simulink model "x1_2_P2_Control_Loop"  (R2021b)
settings: Solver=VariableStepAuto  StartTime=0.0  StopTime=2000  RelTol=1e-3
libraries: slpidlib x2
settings Model: Creator=Edwar  LastModifiedBy=Edwar

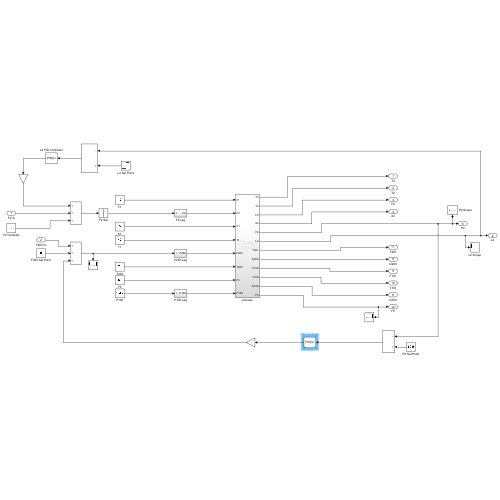
[thumbnail: Simulink's stored preview of the top-level diagram]
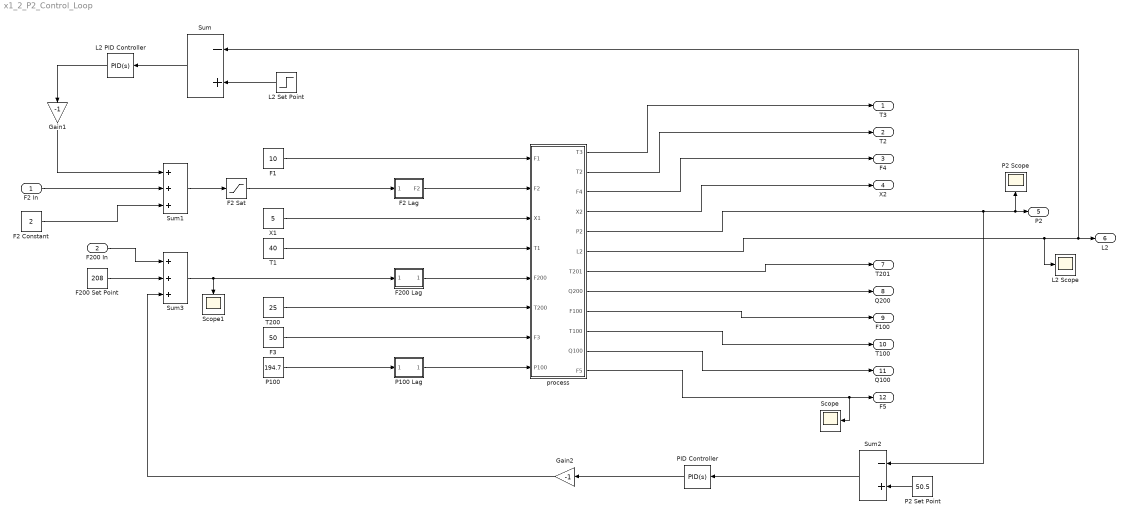
== system x1_2_P2_Control_Loop ==
  F2 In : Inport
  F200 In : Inport  Port=2
  F1 : Constant  Value=10
  F2 Constant : Constant  Value=2
  F2 Lag : Subsystem
  F2 Sat : Saturate  UpperLimit=4  LowerLimit=0
  F200 Lag : Subsystem
  F200 Set Point : Constant  Value=208
  F3 : Constant  Value=50
  Gain1 : Gain  Gain=-1
  Gain2 : Gain  Gain=-1
  L2 PID Controller : slpidlib/PID Controller  Controller=PID  Form=Ideal  TimeDomain=Continuous-time  UseExternalTs=off  SampleTime=-1  IntegratorMethod=Forward Euler  FilterMethod=Forward Euler  ControllerParametersSource=internal  P=14  I=1/19  D=0  UseFilter=on  N=100  TunerSelectOption=Transfer Function Based (PID Tuner App)  InitialConditionSource=internal  InitialConditionForIntegrator=0  InitialConditionForFilter=0  DifferentiatorICPrevScaledInput=0  ExternalReset=none  TrackingMode=off  Kt=1  LimitOutput=off  SatLimitsSource=internal  UpperSaturationLimit=inf  LowerSaturationLimit=-inf  LinearizeAsGain=on  AntiWindupMode=none  Kb=1  POutMin=[]  POutMax=[]  IOutMin=[]  IOutMax=[]  DOutMin=[]  DOutMax=[]  NOutMin=[]  NOutMax=[]  SumOutMin=[]  SumOutMax=[]  SaturationOutMin=[]  SaturationOutMax=[]  PParamMin=[]  PParamMax=[]  IParamMin=[]  IParamMax=[]  DParamMin=[]  DParamMax=[]  NParamMin=[]  NParamMax=[]  KbParamMin=[]  KbParamMax=[]  KtParamMin=[]  KtParamMax=[]  KbOutMin=[]  KbOutMax=[]  KtOutMin=[]  KtOutMax=[]  IntegratorOutMin=[]  IntegratorOutMax=[]  FilterOutMin=[]  FilterOutMax=[]  SumI1OutMin=[]  SumI1OutMax=[]  SumI2OutMin=[]  SumI2OutMax=[]  SumI3OutMin=[]  SumI3OutMax=[]  SumI4OutMin=[]  SumI4OutMax=[]  SumDOutMin=[]  SumDOutMax=[]  DifferentiatorOutMin=[]  DifferentiatorOutMax=[]  FilterDiffOutCoefMin=[]  FilterDiffOutCoefMax=[]  ReciprocalOutMin=[]  ReciprocalOutMax=[]  SumDenOutMin=[]  SumDenOutMax=[]  SumNumOutMin=[]  SumNumOutMax=[]  DivideOutMin=[]  DivideOutMax=[]  UdiffTsProdOutMin=[]  UdiffTsProdOutMax=[]  NTsProdOutMin=[]  NTsProdOutMax=[]  UintegralTsProdOutMin=[]  UintegralTsProdOutMax=[]  UngainTsProdOutMin=[]  UngainTsProdOutMax=[]  IntegratorContinuousStateAttributes=''  IntegratorStateMustResolveToSignalObject=off  IntegratorRTWStateStorageClass=Auto  FilterContinuousStateAttributes=''  FilterStateMustResolveToSignalObject=off  FilterRTWStateStorageClass=Auto  ParallelPVariant=Passthrough  IdealPVariant=InternalParameters  IVariant=InternalParameters  DVariant=InternalParameters  IntegratorVariant=Continuous  SatVariant=Disabled  AWVariant=Passthrough  PCopyVariant=Disabled  TRVariant=Disabled  FdbkBlocksVariant=Forward  IdealPFdbkVariant=Disabled  SatFdbkVariant=Disabled  DerivativeFilterVariant=ContFilter  NVariant=InternalParameters  NCopyVariant=Disabled  FilterICVariant=InternalICsFilter  IntegratorICVariant=InternalICs  ExternalResetVariant=Disabled  TRSumVariant=Passthrough  SumFdbkVariant=Disabled  SumVariant=Sum_PID  TsampFilterVariant=InternalTs  TsampNgainVariant=Passthrough  TsampIntegralVariant=Passthrough  ExternalSaturationOutDataTypeStr=Inherit: Same as second input
  L2 Scope : Scope
  L2 Set Point : Step  Time=1000  Before=1  SampleTime=0
  P100 : Constant  Value=194.7
  P100 Lag : Subsystem
  P2 Scope : Scope
  P2 Set Point : Constant  Value=50.5
  PID Controller : slpidlib/PID Controller  Controller=PID  Form=Ideal  TimeDomain=Continuous-time  UseExternalTs=off  SampleTime=-1  IntegratorMethod=Forward Euler  FilterMethod=Forward Euler  ControllerParametersSource=internal  P=5  I=1  D=0  UseFilter=on  N=100  TunerSelectOption=Transfer Function Based (PID Tuner App)  InitialConditionSource=internal  InitialConditionForIntegrator=0  InitialConditionForFilter=0  DifferentiatorICPrevScaledInput=0  ExternalReset=none  TrackingMode=off  Kt=1  LimitOutput=off  SatLimitsSource=internal  UpperSaturationLimit=inf  LowerSaturationLimit=-inf  LinearizeAsGain=on  AntiWindupMode=none  Kb=1  POutMin=[]  POutMax=[]  IOutMin=[]  IOutMax=[]  DOutMin=[]  DOutMax=[]  NOutMin=[]  NOutMax=[]  SumOutMin=[]  SumOutMax=[]  SaturationOutMin=[]  SaturationOutMax=[]  PParamMin=[]  PParamMax=[]  IParamMin=[]  IParamMax=[]  DParamMin=[]  DParamMax=[]  NParamMin=[]  NParamMax=[]  KbParamMin=[]  KbParamMax=[]  KtParamMin=[]  KtParamMax=[]  KbOutMin=[]  KbOutMax=[]  KtOutMin=[]  KtOutMax=[]  IntegratorOutMin=[]  IntegratorOutMax=[]  FilterOutMin=[]  FilterOutMax=[]  SumI1OutMin=[]  SumI1OutMax=[]  SumI2OutMin=[]  SumI2OutMax=[]  SumI3OutMin=[]  SumI3OutMax=[]  SumI4OutMin=[]  SumI4OutMax=[]  SumDOutMin=[]  SumDOutMax=[]  DifferentiatorOutMin=[]  DifferentiatorOutMax=[]  FilterDiffOutCoefMin=[]  FilterDiffOutCoefMax=[]  ReciprocalOutMin=[]  ReciprocalOutMax=[]  SumDenOutMin=[]  SumDenOutMax=[]  SumNumOutMin=[]  SumNumOutMax=[]  DivideOutMin=[]  DivideOutMax=[]  UdiffTsProdOutMin=[]  UdiffTsProdOutMax=[]  NTsProdOutMin=[]  NTsProdOutMax=[]  UintegralTsProdOutMin=[]  UintegralTsProdOutMax=[]  UngainTsProdOutMin=[]  UngainTsProdOutMax=[]  IntegratorContinuousStateAttributes=''  IntegratorStateMustResolveToSignalObject=off  IntegratorRTWStateStorageClass=Auto  FilterContinuousStateAttributes=''  FilterStateMustResolveToSignalObject=off  FilterRTWStateStorageClass=Auto  ParallelPVariant=Passthrough  IdealPVariant=InternalParameters  IVariant=InternalParameters  DVariant=InternalParameters  IntegratorVariant=Continuous  SatVariant=Disabled  AWVariant=Passthrough  PCopyVariant=Disabled  TRVariant=Disabled  FdbkBlocksVariant=Forward  IdealPFdbkVariant=Disabled  SatFdbkVariant=Disabled  DerivativeFilterVariant=ContFilter  NVariant=InternalParameters  NCopyVariant=Disabled  FilterICVariant=InternalICsFilter  IntegratorICVariant=InternalICs  ExternalResetVariant=Disabled  TRSumVariant=Passthrough  SumFdbkVariant=Disabled  SumVariant=Sum_PID  TsampFilterVariant=InternalTs  TsampNgainVariant=Passthrough  TsampIntegralVariant=Passthrough  ExternalSaturationOutDataTypeStr=Inherit: Same as second input
  Scope : Scope
  Scope1 : Scope
  Sum : Sum  Inputs=-+
  Sum1 : Sum  Inputs=+++
  Sum2 : Sum  Inputs=-+
  Sum3 : Sum  Inputs=+++
  T1 : Constant  Value=40
  T200 : Constant  Value=25
  X1 : Constant  Value=5
  process : Subsystem
  T3 : Outport
  T2 : Outport  Port=2
  F4 : Outport  Port=3
  X2 : Outport  Port=4
  P2 : Outport  Port=5
  L2 : Outport  Port=6
  T201 : Outport  Port=7
  Q200 : Outport  Port=8
  F100 : Outport  Port=9
  T100 : Outport  Port=10
  Q100 : Outport  Port=11
  F5 : Outport  Port=12
  wires:
  Gain1/1 -> Sum1/1
  Sum/1 -> L2 PID Controller/1
  F2 In/1 -> Sum1/2
  F2 Lag/1(F2) -> process/2(F2)
  T200/1 -> process/6(T200)
  F2 Sat/1 -> F2 Lag/1(1)
  Sum3/1 -> F200 Lag/1(1), Scope1/1
  process/4(X2) -> X2/1
  Sum1/1 -> F2 Sat/1
  process/9(F100) -> F100/1
  process/1(T3) -> T3/1
  process/7(T201) -> T201/1
  P100 Lag/1(P100) -> process/8(P100)
  F200 Lag/1(F200) -> process/5(F200)
  L2 Set Point/1 -> Sum/2
  P100/1 -> P100 Lag/1(1)
  process/2(T2) -> T2/1
  process/10(T100) -> T100/1
  T1/1 -> process/4(T1)
  process/3(F4) -> F4/1
  F3/1 -> process/7(F3)
  process/5(P2) -> Sum2/1, P2 Scope/1, P2/1
  process/11(Q100) -> Q100/1
  L2 PID Controller/1 -> Gain1/1
  F2 Constant/1 -> Sum1/3
  process/6(L2) -> L2 Scope/1, Sum/1, L2/1
  process/8(Q200) -> Q200/1
  process/12(F5) -> Scope/1, F5/1
  P2 Set Point/1 -> Sum2/2
  Sum2/1 -> PID Controller/1
  PID Controller/1 -> Gain2/1
  F200 In/1 -> Sum3/1
  F200 Set Point/1 -> Sum3/2
  Gain2/1 -> Sum3/3
  F1/1 -> process/1(F1)
  X1/1 -> process/3(X1)

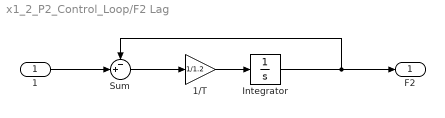
== system x1_2_P2_Control_Loop/F2 Lag ==
  1 : Inport
  1/T : Gain  Gain=1/1.2
  Integrator : Integrator  InitialCondition=2
  Sum : Sum  Inputs=-+|
  F2 : Outport
  wires:
  Integrator/1 -> F2/1, Sum/1
  Sum/1 -> 1/T/1
  1/T/1 -> Integrator/1
  1/1 -> Sum/2

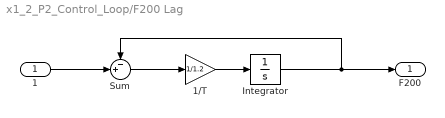
== system x1_2_P2_Control_Loop/F200 Lag ==
  1 : Inport
  1/T : Gain  Gain=1/1.2
  Integrator : Integrator  InitialCondition=208
  Sum : Sum  Inputs=-+|
  F200 : Outport
  wires:
  Integrator/1 -> F200/1, Sum/1
  Sum/1 -> 1/T/1
  1/T/1 -> Integrator/1
  1/1 -> Sum/2

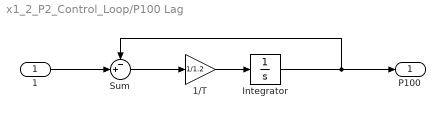
== system x1_2_P2_Control_Loop/P100 Lag ==
  1 : Inport
  1/T : Gain  Gain=1/1.2
  Integrator : Integrator  InitialCondition=194.7
  Sum : Sum  Inputs=-+|
  P100 : Outport
  wires:
  Integrator/1 -> P100/1, Sum/1
  Sum/1 -> 1/T/1
  1/T/1 -> Integrator/1
  1/1 -> Sum/2

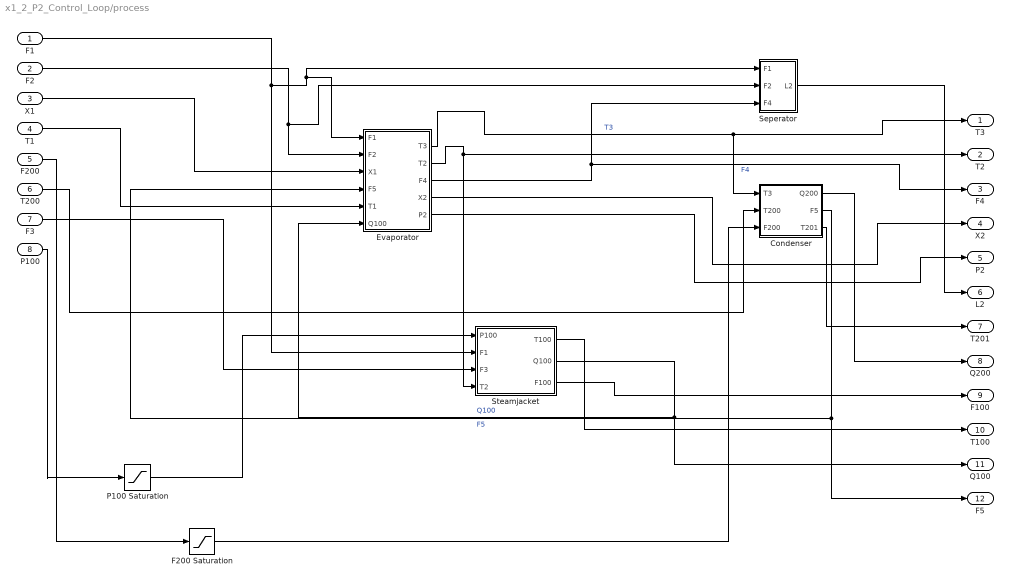
== system x1_2_P2_Control_Loop/process ==
  F1 : Inport
  F2 : Inport  Port=2
  X1 : Inport  Port=3
  T1 : Inport  Port=4
  F200 : Inport  Port=5
  T200 : Inport  Port=6
  F3 : Inport  Port=7
  P100 : Inport  Port=8
  Condenser : Subsystem
  Evaporator : Subsystem
  F200 Saturation : Saturate  UpperLimit=416  LowerLimit=0
  P100 Saturation : Saturate  UpperLimit=400  LowerLimit=0
  Seperator : Subsystem
  Steamjacket : Subsystem
  T3 : Outport
  T2 : Outport  Port=2
  F4 : Outport  Port=3
  X2 : Outport  Port=4
  P2 : Outport  Port=5
  L2 : Outport  Port=6
  T201 : Outport  Port=7
  Q200 : Outport  Port=8
  F100 : Outport  Port=9
  T100 : Outport  Port=10
  Q100 : Outport  Port=11
  F5 : Outport  Port=12
  wires:
  P100 Saturation/1 -> Steamjacket/1(P100)
  F200 Saturation/1 -> Condenser/3(F200)
  Condenser/1(Q200) -> Q200/1
  T200/1 -> Condenser/2(T200)
  T1/1 -> Evaporator/5(T1)
  Seperator/1(L2) -> L2/1
  Steamjacket/3(F100) -> F100/1
  Steamjacket/1(T100) -> T100/1
  Evaporator/5(P2) -> P2/1
  P100/1 -> P100 Saturation/1
  F3/1 -> Steamjacket/3(F3)
  Condenser/3(T201) -> T201/1
  Steamjacket/2(Q100) -> Evaporator/6(Q100), Q100/1  "Q100"
  X1/1 -> Evaporator/3(X1)
  Evaporator/4(X2) -> X2/1
  Evaporator/1(T3) -> Condenser/1(T3), T3/1  "T3"
  Evaporator/3(F4) -> Seperator/3(F4), F4/1  "F4"
  F200/1 -> F200 Saturation/1
  F1/1 -> Evaporator/1(F1), Seperator/1(F1), Steamjacket/2(F1)
  Evaporator/2(T2) -> Steamjacket/4(T2), T2/1
  Condenser/2(F5) -> Evaporator/4(F5), F5/1  "F5"
  F2/1 -> Evaporator/2(F2), Seperator/2(F2)

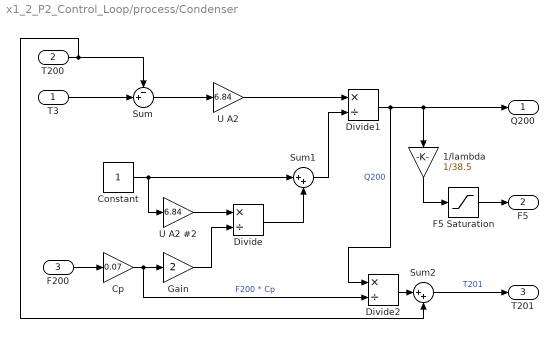
== system x1_2_P2_Control_Loop/process/Condenser ==
  T3 : Inport
  T200 : Inport  Port=2
  F200 : Inport  Port=3
  1/lambda : Gain  Gain=1/38.5
  Constant : Constant
  Cp : Gain  Gain=0.07
  Divide : Product  Inputs=*/
  Divide1 : Product  Inputs=*/
  Divide2 : Product  Inputs=*/
  F5 Saturation : Saturate  UpperLimit=16  LowerLimit=0
  Gain : Gain  Gain=2
  Sum : Sum  Inputs=-+|
  Sum1 : Sum  Inputs=|++
  Sum2 : Sum  Inputs=|++
  U A2 : Gain  Gain=6.84
  U A2 #2 : Gain  Gain=6.84
  Q200 : Outport
  F5 : Outport  Port=2
  T201 : Outport  Port=3
  wires:
  F5 Saturation/1 -> F5/1
  1/lambda/1 -> F5 Saturation/1
  Divide2/1 -> Sum2/1
  Sum2/1 -> T201/1  "T201"
  Cp/1 -> Gain/1, Divide2/2  "F200 * Cp"
  U A2 #2/1 -> Divide/1
  T3/1 -> Sum/2
  Constant/1 -> Sum1/1, U A2 #2/1
  Sum/1 -> U A2/1
  F200/1 -> Cp/1
  U A2/1 -> Divide1/1
  Divide1/1 -> 1/lambda/1, Q200/1, Divide2/1  "Q200"
  Divide/1 -> Sum1/2
  T200/1 -> Sum/1, Sum2/2
  Gain/1 -> Divide/2
  Sum1/1 -> Divide1/2

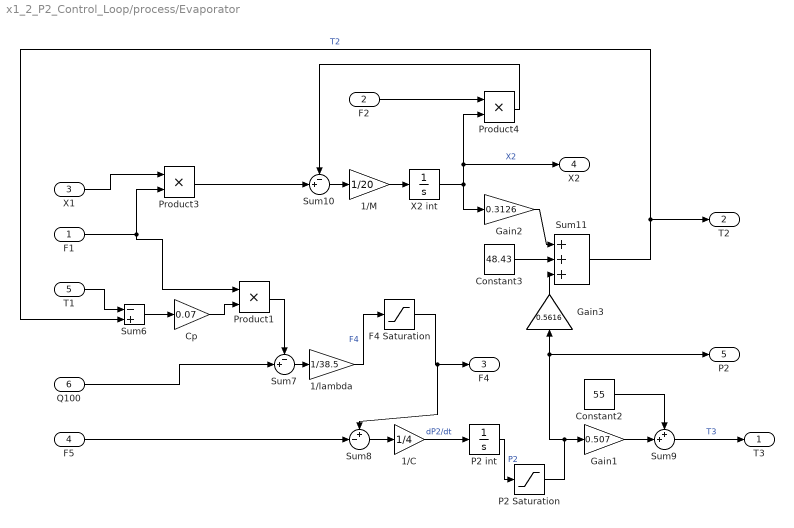
== system x1_2_P2_Control_Loop/process/Evaporator ==
  F1 : Inport
  F2 : Inport  Port=2
  X1 : Inport  Port=3
  F5 : Inport  Port=4
  T1 : Inport  Port=5
  Q100 : Inport  Port=6
  1/C : Gain  Gain=1/4
  1/M : Gain  Gain=1/20
  1/lambda : Gain  Gain=1/38.5
  Constant2 : Constant  Value=55
  Constant3 : Constant  Value=48.43
  Cp : Gain  Gain=0.07
  F4 Saturation : Saturate  UpperLimit=16  LowerLimit=0
  Gain1 : Gain  Gain=0.507
  Gain2 : Gain  Gain=0.3126
  Gain3 : Gain  Gain=0.5616
  P2 Saturation : Saturate  UpperLimit=100  LowerLimit=0
  P2 int : Integrator  InitialCondition=50.5
  Product1 : Product
  Product3 : Product
  Product4 : Product
  Sum10 : Sum  Inputs=-+|
  Sum11 : Sum  Inputs=+++
  Sum6 : Sum  Inputs=-+
  Sum7 : Sum  Inputs=-+|
  Sum8 : Sum  Inputs=+-|
  Sum9 : Sum  Inputs=++|
  X2 int : Integrator  InitialCondition=25
  T3 : Outport
  T2 : Outport  Port=2
  F4 : Outport  Port=3
  X2 : Outport  Port=4
  P2 : Outport  Port=5
  wires:
  P2 Saturation/1 -> Gain1/1, Gain3/1, P2/1
  F4 Saturation/1 -> F4/1, Sum8/1
  1/lambda/1 -> F4 Saturation/1  "F4"
  F5/1 -> Sum8/2
  X1/1 -> Product3/1
  T1/1 -> Sum6/1
  Cp/1 -> Product1/2
  Product4/1 -> Sum10/1
  Sum10/1 -> 1/M/1
  P2 int/1 -> P2 Saturation/1  "P2"
  Sum8/1 -> 1/C/1
  Sum6/1 -> Cp/1
  Gain1/1 -> Sum9/2
  F1/1 -> Product3/2, Product1/1
  Product1/1 -> Sum7/1
  Product3/1 -> Sum10/2
  Sum7/1 -> 1/lambda/1
  Sum11/1 -> Sum6/2, T2/1  "T2"
  X2 int/1 -> Gain2/1, Product4/2, X2/1  "X2"
  Q100/1 -> Sum7/2
  Constant2/1 -> Sum9/1
  Gain2/1 -> Sum11/1
  Constant3/1 -> Sum11/2
  Gain3/1 -> Sum11/3
  1/M/1 -> X2 int/1
  Sum9/1 -> T3/1  "T3"
  1/C/1 -> P2 int/1  "dP2/dt"
  F2/1 -> Product4/1

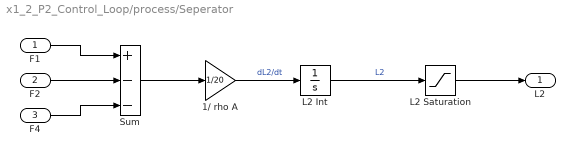
== system x1_2_P2_Control_Loop/process/Seperator ==
  F1 : Inport
  F2 : Inport  Port=2
  F4 : Inport  Port=3
  1/ rho A : Gain  Gain=1/20
  L2 Int : Integrator  InitialCondition=1
  L2 Saturation : Saturate  UpperLimit=2  LowerLimit=0
  Sum : Sum  Inputs=+--
  L2 : Outport
  wires:
  L2 Saturation/1 -> L2/1
  F1/1 -> Sum/1
  1/ rho A/1 -> L2 Int/1  "dL2/dt"
  F2/1 -> Sum/2
  F4/1 -> Sum/3
  L2 Int/1 -> L2 Saturation/1  "L2"
  Sum/1 -> 1/ rho A/1

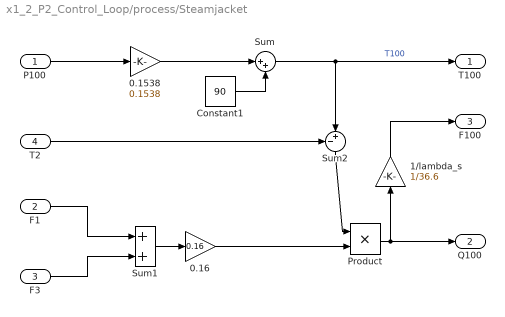
== system x1_2_P2_Control_Loop/process/Steamjacket ==
  P100 : Inport
  F1 : Inport  Port=2
  F3 : Inport  Port=3
  T2 : Inport  Port=4
  0.1538 : Gain  Gain=0.1538
  0.16 : Gain  Gain=0.16
  1/lambda_s : Gain  Gain=1/36.6
  Constant1 : Constant  Value=90
  Product : Product
  Sum : Sum  Inputs=|++
  Sum1 : Sum
  Sum2 : Sum  Inputs=-+|
  T100 : Outport
  Q100 : Outport  Port=2
  F100 : Outport  Port=3
  wires:
  F3/1 -> Sum1/2
  0.16/1 -> Product/2
  Sum1/1 -> 0.16/1
  P100/1 -> 0.1538/1
  F1/1 -> Sum1/1
  Sum/1 -> Sum2/2, T100/1  "T100"
  Sum2/1 -> Product/1
  0.1538/1 -> Sum/1
  Product/1 -> 1/lambda_s/1, Q100/1
  T2/1 -> Sum2/1
  1/lambda_s/1 -> F100/1
  Constant1/1 -> Sum/2
